simulink model "SIMULACIONT1P1"  (R2022b)
settings: Solver=VariableStepAuto  StartTime=0.0  StopTime=12  RelTol=1e-3
settings Model: Creator=David  LastModifiedBy=David

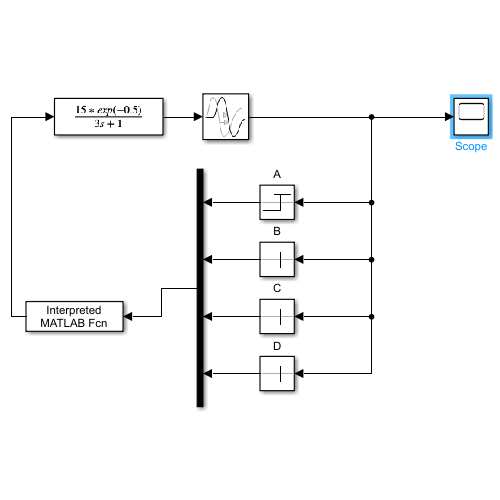
[thumbnail: Simulink's stored preview of the top-level diagram]
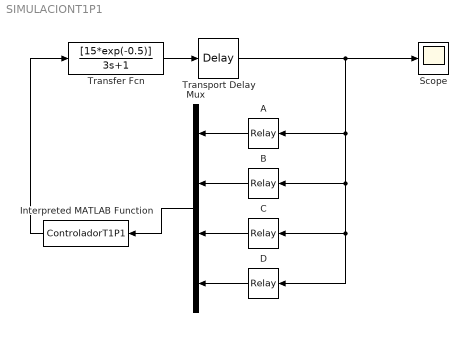
== system SIMULACIONT1P1 ==
  A : Relay  OnSwitchValue=1  OffSwitchValue=1
  B : Relay  OnSwitchValue=0.75  OffSwitchValue=0.75
  C : Relay  OnSwitchValue=0.5  OffSwitchValue=0.5
  D : Relay  OnSwitchValue=0.25  OffSwitchValue=0.25
  Interpreted MATLAB Function : MATLABFcn  MATLABFcn=ControladorT1P1  OutputDimensions=1
  Mux : Mux
  Scope : Scope
  Transfer Fcn : TransferFcn  Numerator=[15*exp(-0.5)]  Denominator=[3 1]
  Transport Delay : TransportDelay  DelayTime=0.5
  wires:
  Mux/1 -> Interpreted MATLAB Function/1
  Transfer Fcn/1 -> Transport Delay/1
  A/1 -> Mux/1
  B/1 -> Mux/2
  C/1 -> Mux/3
  D/1 -> Mux/4
  Transport Delay/1 -> D/1, C/1, B/1, A/1, Scope/1
  Interpreted MATLAB Function/1 -> Transfer Fcn/1
